simulink model "Simulink_generic_interface_2018b"  (R2018b)
settings: Solver=FixedStepAuto  StartTime=0.0  StopTime=inf  FixedStep=0.0005  RelTol=1e-3
settings Model: Creator=matti  LastModifiedBy=User
settings DataIOCC: ReturnWorkspaceOutputs=on
settings DebuggingCC: UnconnectedInputMsg=none  UnconnectedOutputMsg=none  UnconnectedLineMsg=none
settings ModelReferenceCC: EnableRefExpFcnMdlSchedulingChecks=off
settings RTWCC: Description=Generic Real-Time Target

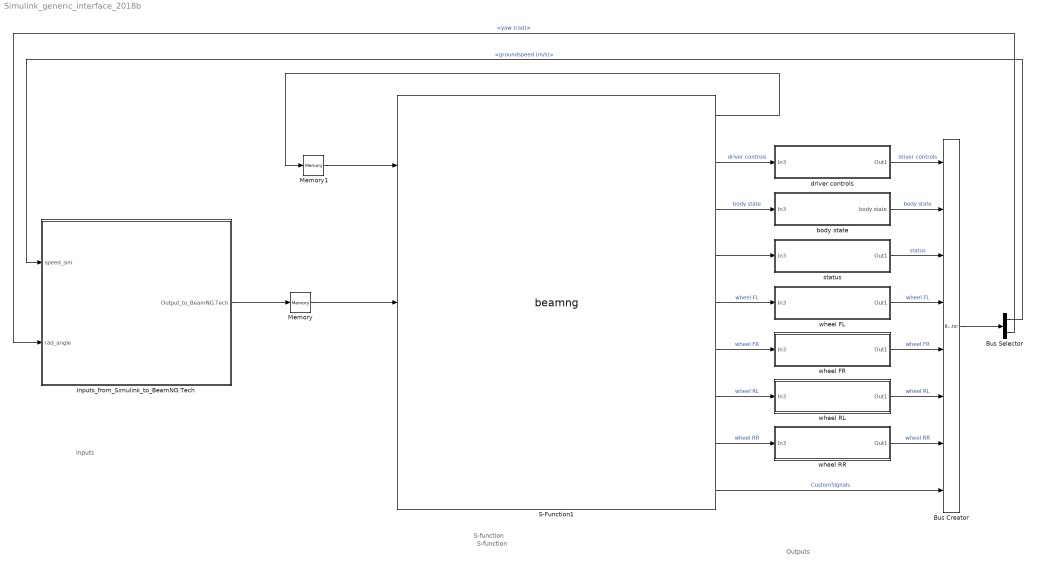
== system Simulink_generic_interface_2018b ==
  note: Inputs
  note: S-function
  note: S-function
  note: Outputs
  Bus Creator : BusCreator  Inputs=8
  Bus Selector : BusSelector  OutputSignals=body state.groundspeed (m/s),body state.yaw (rad)
  Inputs_from_Simulink_to_BeamNG.Tech : Subsystem
  Memory : Memory
  Memory1 : Memory
  S-Function1 : S-Function  FunctionName=beamng  SFunctionDeploymentMode=off  EnableBusSupport=off
      mask Display: image('logo_beamng1.png')
  body state : Subsystem
  driver controls : Subsystem
  status : Subsystem
  wheel FL : Subsystem
  wheel FR : Subsystem
  wheel RL : Subsystem
  wheel RR : Subsystem
  wires:
  S-Function1/3 -> body state/1(In3)  "body state"
  S-Function1/9 -> Bus Creator/8  "CustomSignals"
  S-Function1/5 -> wheel FL/1(In3)  "wheel FL"
  S-Function1/6 -> wheel FR/1(In3)  "wheel FR"
  S-Function1/7 -> wheel RL/1(In3)  "wheel RL"
  S-Function1/8 -> wheel RR/1(In3)  "wheel RR"
  S-Function1/2 -> driver controls/1(In3)  "driver controls"
  Bus Creator/1 -> Bus Selector/1
  Bus Selector/1 -> Inputs_from_Simulink_to_BeamNG.Tech/1(speed_sim)  "<groundspeed (m/s)>"
  Bus Selector/2 -> Inputs_from_Simulink_to_BeamNG.Tech/2(rad_angle)  "<yaw (rad)>"
  driver controls/1(Out1) -> Bus Creator/1  "driver controls"
  body state/1(body state) -> Bus Creator/2  "body state"
  status/1(Out1) -> Bus Creator/3  "status"
  wheel FL/1(Out1) -> Bus Creator/4  "wheel FL"
  wheel FR/1(Out1) -> Bus Creator/5  "wheel FR"
  wheel RL/1(Out1) -> Bus Creator/6  "wheel RL"
  wheel RR/1(Out1) -> Bus Creator/7  "wheel RR"
  Memory/1 -> S-Function1/2
  Inputs_from_Simulink_to_BeamNG.Tech/1(Output_to_BeamNG.Tech) -> Memory/1
  Memory1/1 -> S-Function1/1
  S-Function1/1 -> Memory1/1
  S-Function1/4 -> status/1(In3)

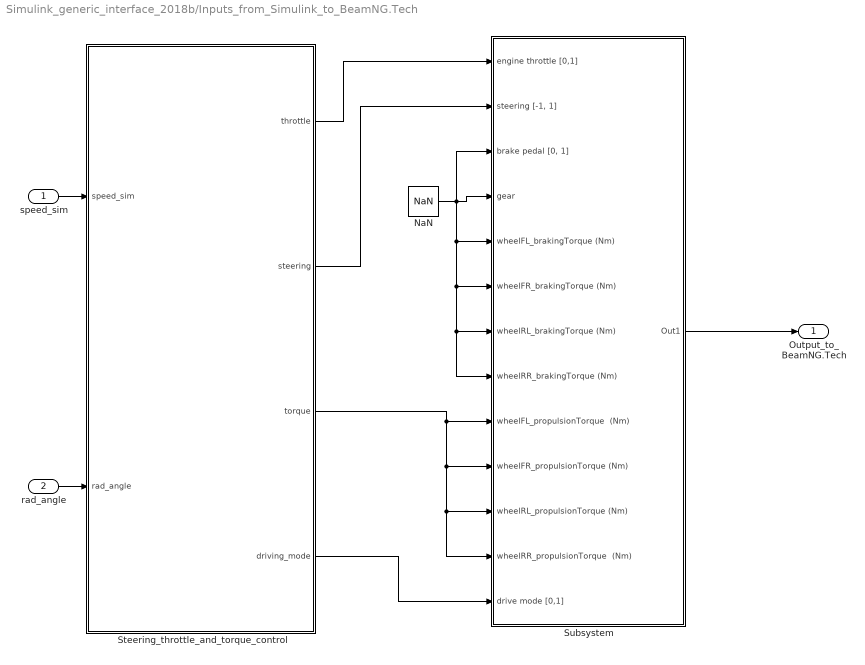
== system Simulink_generic_interface_2018b/Inputs_from_Simulink_to_BeamNG.Tech ==
  speed_sim : Inport
  rad_angle : Inport  Port=2
  NaN : Constant  Value=NaN  OutDataTypeStr=Inherit: Inherit via back propagation
  Steering_throttle_and_torque_control : Subsystem
  Subsystem : Subsystem
  Output_to_BeamNG.Tech : Outport  VectorParamsAs1DForOutWhenUnconnected=on
  wires:
  rad_angle/1 -> Steering_throttle_and_torque_control/2(rad_angle)
  Subsystem/1(Out1) -> Output_to_BeamNG.Tech/1
  speed_sim/1 -> Steering_throttle_and_torque_control/1(speed_sim)
  Steering_throttle_and_torque_control/3(torque) -> Subsystem/10(wheelFR_propulsionTorque (Nm)), Subsystem/11(wheelRL_propulsionTorque (Nm)), Subsystem/12(wheelRR_propulsionTorque	 (Nm)), Subsystem/9(wheelFL_propulsionTorque	 (Nm))
  Steering_throttle_and_torque_control/4(driving_mode) -> Subsystem/13(drive mode [0,1])
  Steering_throttle_and_torque_control/2(steering) -> Subsystem/2("steering\t[-1, 1]")
  Steering_throttle_and_torque_control/1(throttle) -> Subsystem/1("engine throttle [0,1] ")
  NaN/1 -> Subsystem/3("brake pedal [0, 1]"), Subsystem/8("wheelRR_brakingTorque (Nm)\t"), Subsystem/7("wheelRL_brakingTorque (Nm)\t"), Subsystem/6("wheelFR_brakingTorque (Nm)\t"), Subsystem/5("wheelFL_brakingTorque (Nm)\t"), Subsystem/4("gear ")

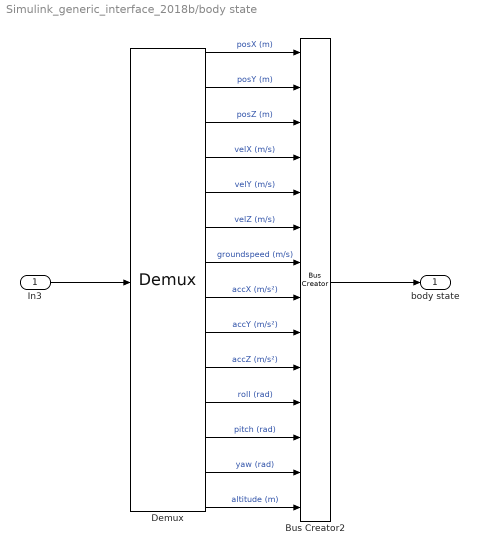
== system Simulink_generic_interface_2018b/body state ==
  In3 : Inport
  Bus Creator2 : BusCreator  Inputs=14
  Demux : Demux  Outputs=14
  body state : Outport  VectorParamsAs1DForOutWhenUnconnected=on
  wires:
  In3/1 -> Demux/1
  Demux/1 -> Bus Creator2/1  "posX (m)"
  Demux/2 -> Bus Creator2/2  "posY (m)"
  Demux/3 -> Bus Creator2/3  "posZ (m)"
  Demux/4 -> Bus Creator2/4  "velX (m/s)"
  Demux/5 -> Bus Creator2/5  "velY (m/s)"
  Demux/6 -> Bus Creator2/6  "velZ (m/s)"
  Demux/7 -> Bus Creator2/7  "groundspeed (m/s)"
  Demux/8 -> Bus Creator2/8  "accX (m/s²)"
  Demux/9 -> Bus Creator2/9  "accY (m/s²)"
  Demux/10 -> Bus Creator2/10  "accZ (m/s²)"
  Demux/11 -> Bus Creator2/11  "roll (rad)"
  Demux/12 -> Bus Creator2/12  "pitch (rad)"
  Demux/13 -> Bus Creator2/13  "yaw (rad)"
  Demux/14 -> Bus Creator2/14  "altitude (m)"
  Bus Creator2/1 -> body state/1

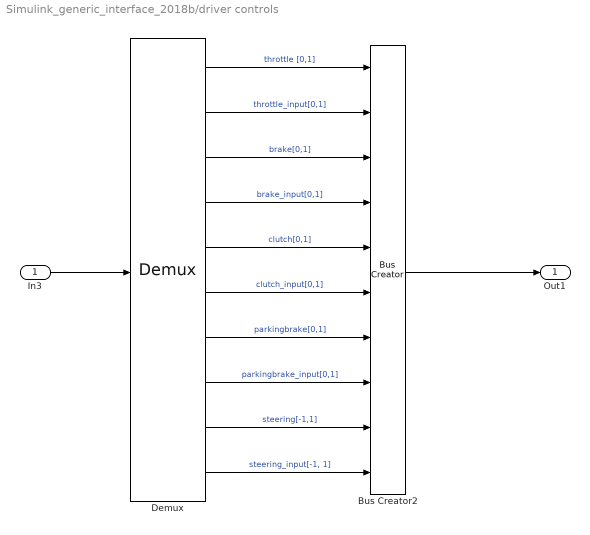
== system Simulink_generic_interface_2018b/driver controls ==
  In3 : Inport
  Bus Creator2 : BusCreator  Inputs=10
  Demux : Demux  Outputs=10
  Out1 : Outport  VectorParamsAs1DForOutWhenUnconnected=on
  wires:
  In3/1 -> Demux/1
  Demux/1 -> Bus Creator2/1  "throttle [0,1]"
  Demux/2 -> Bus Creator2/2  "throttle_input[0,1]"
  Demux/3 -> Bus Creator2/3  "brake[0,1]"
  Demux/4 -> Bus Creator2/4  "brake_input[0,1]"
  Demux/5 -> Bus Creator2/5  "clutch[0,1]"
  Demux/6 -> Bus Creator2/6  "clutch_input[0,1]"
  Demux/7 -> Bus Creator2/7  "parkingbrake[0,1]"
  Demux/8 -> Bus Creator2/8  "parkingbrake_input[0,1]"
  Demux/9 -> Bus Creator2/9  "steering[-1,1]"
  Demux/10 -> Bus Creator2/10  "steering_input[-1, 1]"
  Bus Creator2/1 -> Out1/1

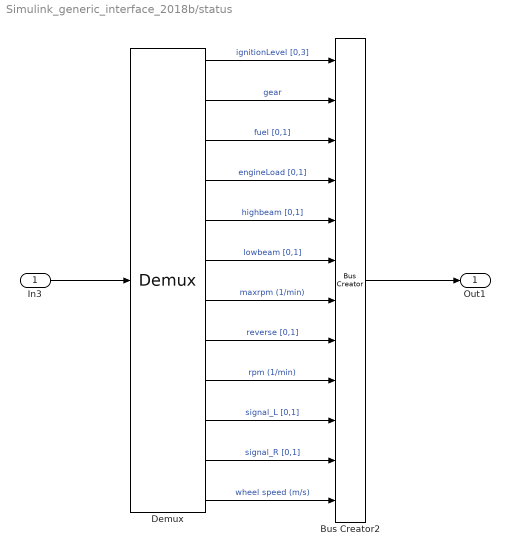
== system Simulink_generic_interface_2018b/status ==
  In3 : Inport
  Bus Creator2 : BusCreator  Inputs=12
  Demux : Demux  Outputs=12
  Out1 : Outport  VectorParamsAs1DForOutWhenUnconnected=on
  wires:
  Demux/12 -> Bus Creator2/12  "wheel speed (m/s)"
  Demux/11 -> Bus Creator2/11  "signal_R [0,1]"
  Demux/10 -> Bus Creator2/10  "signal_L [0,1]"
  Demux/9 -> Bus Creator2/9  "rpm (1/min)"
  Demux/8 -> Bus Creator2/8  "reverse [0,1]"
  Demux/7 -> Bus Creator2/7  "maxrpm (1/min)"
  Demux/6 -> Bus Creator2/6  "lowbeam [0,1]"
  Demux/5 -> Bus Creator2/5  "highbeam [0,1]"
  Demux/4 -> Bus Creator2/4  "engineLoad [0,1]"
  Demux/3 -> Bus Creator2/3  "fuel [0,1]"
  Demux/2 -> Bus Creator2/2  "gear"
  Demux/1 -> Bus Creator2/1  "ignitionLevel [0,3]"
  In3/1 -> Demux/1
  Bus Creator2/1 -> Out1/1

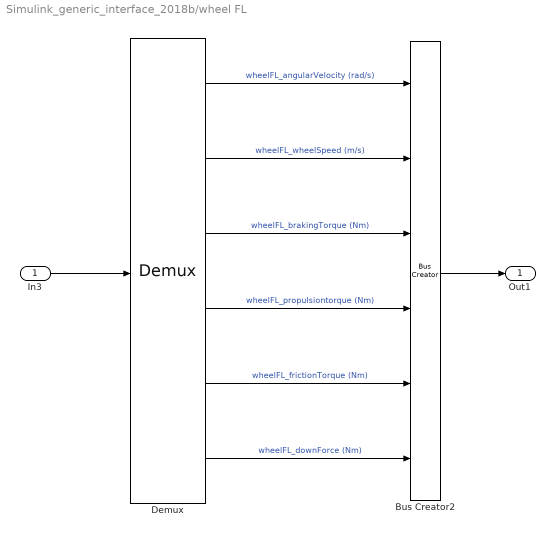
== system Simulink_generic_interface_2018b/wheel FL ==
  In3 : Inport
  Bus Creator2 : BusCreator  Inputs=6
  Demux : Demux  Outputs=6
  Out1 : Outport  VectorParamsAs1DForOutWhenUnconnected=on
  wires:
  In3/1 -> Demux/1
  Demux/1 -> Bus Creator2/1  "wheelFL_angularVelocity (rad/s)"
  Demux/2 -> Bus Creator2/2  "wheelFL_wheelSpeed (m/s)"
  Demux/3 -> Bus Creator2/3  "wheelFL_brakingTorque (Nm)"
  Demux/4 -> Bus Creator2/4  "wheelFL_propulsiontorque (Nm)"
  Demux/5 -> Bus Creator2/5  "wheelFL_frictionTorque (Nm)"
  Demux/6 -> Bus Creator2/6  "wheelFL_downForce (Nm)"
  Bus Creator2/1 -> Out1/1

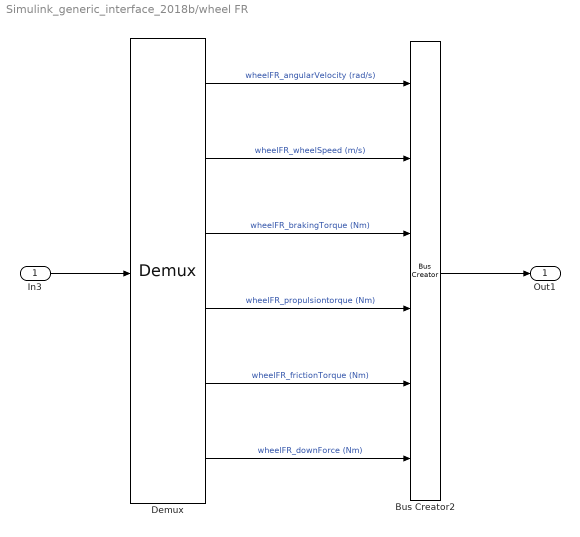
== system Simulink_generic_interface_2018b/wheel FR ==
  In3 : Inport
  Bus Creator2 : BusCreator  Inputs=6
  Demux : Demux  Outputs=6
  Out1 : Outport  VectorParamsAs1DForOutWhenUnconnected=on
  wires:
  Demux/6 -> Bus Creator2/6  "wheelFR_downForce (Nm)"
  Demux/5 -> Bus Creator2/5  "wheelFR_frictionTorque (Nm)"
  Demux/4 -> Bus Creator2/4  "wheelFR_propulsiontorque (Nm)"
  Demux/3 -> Bus Creator2/3  "wheelFR_brakingTorque (Nm)"
  Demux/2 -> Bus Creator2/2  "wheelFR_wheelSpeed (m/s)"
  Demux/1 -> Bus Creator2/1  "wheelFR_angularVelocity (rad/s)"
  In3/1 -> Demux/1
  Bus Creator2/1 -> Out1/1

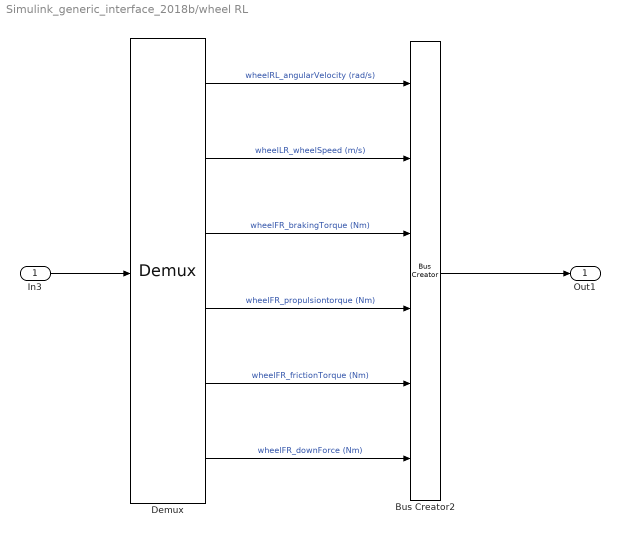
== system Simulink_generic_interface_2018b/wheel RL ==
  In3 : Inport
  Bus Creator2 : BusCreator  Inputs=6
  Demux : Demux  Outputs=6
  Out1 : Outport  VectorParamsAs1DForOutWhenUnconnected=on
  wires:
  In3/1 -> Demux/1
  Demux/1 -> Bus Creator2/1  "wheelRL_angularVelocity (rad/s)"
  Demux/2 -> Bus Creator2/2  "wheelLR_wheelSpeed (m/s)"
  Demux/3 -> Bus Creator2/3  "wheelFR_brakingTorque (Nm)"
  Demux/4 -> Bus Creator2/4  "wheelFR_propulsiontorque (Nm)"
  Demux/5 -> Bus Creator2/5  "wheelFR_frictionTorque (Nm)"
  Demux/6 -> Bus Creator2/6  "wheelFR_downForce (Nm)"
  Bus Creator2/1 -> Out1/1

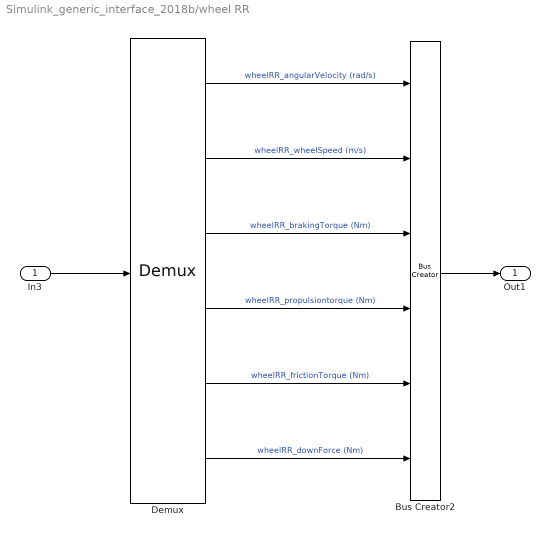
== system Simulink_generic_interface_2018b/wheel RR ==
  In3 : Inport
  Bus Creator2 : BusCreator  Inputs=6
  Demux : Demux  Outputs=6
  Out1 : Outport  VectorParamsAs1DForOutWhenUnconnected=on
  wires:
  Demux/6 -> Bus Creator2/6  "wheelRR_downForce (Nm)"
  Demux/5 -> Bus Creator2/5  "wheelRR_frictionTorque (Nm)"
  Demux/4 -> Bus Creator2/4  "wheelRR_propulsiontorque (Nm)"
  Demux/3 -> Bus Creator2/3  "wheelRR_brakingTorque (Nm)"
  Demux/2 -> Bus Creator2/2  "wheelRR_wheelSpeed (m/s)"
  Demux/1 -> Bus Creator2/1  "wheelRR_angularVelocity (rad/s)"
  In3/1 -> Demux/1
  Bus Creator2/1 -> Out1/1

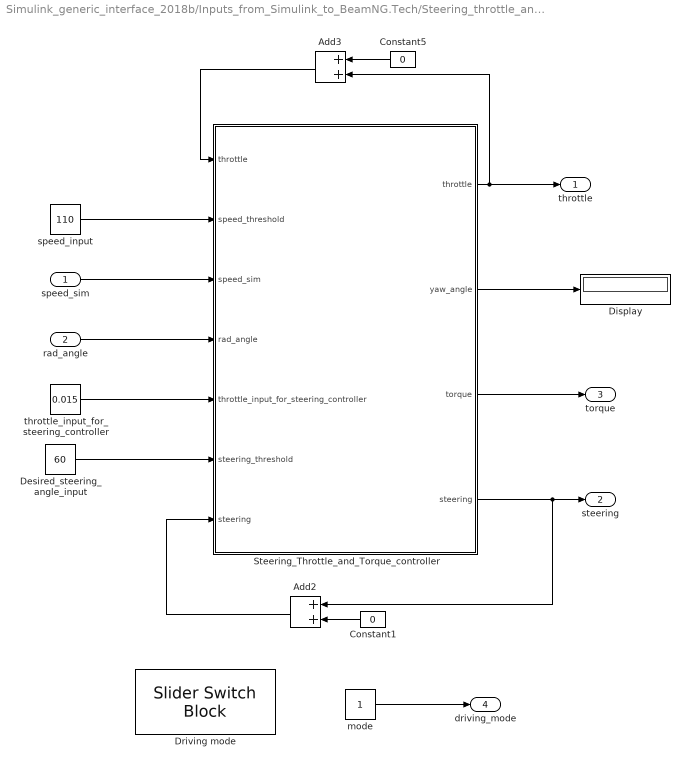
== system Simulink_generic_interface_2018b/Inputs_from_Simulink_to_BeamNG.Tech/Steering_throttle_and_torque_control ==
  speed_sim : Inport
  rad_angle : Inport  Port=2
  Add2 : Sum
  Add3 : Sum
  Constant1 : Constant  Value=0
  Constant5 : Constant  Value=0
  Desired_steering_angle_input : Constant  Value=60
  Display : Display
  Driving mode : SliderSwitchBlock  WebBlockId=467
      settings: Values={{'Torque', 'Pedal'}, [1 0]}
  Steering_Throttle_and_Torque_controller : MATLAB Function  TreatAsAtomicUnit=on
  mode : Constant
  speed_input : Constant  Value=110
  throttle_input_for_steering_controller : Constant  Value=0.015
  throttle : Outport  VectorParamsAs1DForOutWhenUnconnected=on
  steering : Outport  Port=2  VectorParamsAs1DForOutWhenUnconnected=on
  torque : Outport  Port=3  VectorParamsAs1DForOutWhenUnconnected=on
  driving_mode : Outport  Port=4  VectorParamsAs1DForOutWhenUnconnected=on
  wires:
  speed_input/1 -> Steering_Throttle_and_Torque_controller/2(speed_threshold)
  Desired_steering_angle_input/1 -> Steering_Throttle_and_Torque_controller/6(steering_threshold)
  Constant5/1 -> Add3/1
  Steering_Throttle_and_Torque_controller/1(throttle) -> Add3/2, throttle/1
  Add2/1 -> Steering_Throttle_and_Torque_controller/7("steering ")
  Constant1/1 -> Add2/2
  Add3/1 -> Steering_Throttle_and_Torque_controller/1("throttle ")
  mode/1 -> driving_mode/1
  Steering_Throttle_and_Torque_controller/3(torque) -> torque/1
  Steering_Throttle_and_Torque_controller/4(steering) -> Add2/1, steering/1
  rad_angle/1 -> Steering_Throttle_and_Torque_controller/4(rad_angle)
  speed_sim/1 -> Steering_Throttle_and_Torque_controller/3(speed_sim)
  throttle_input_for_steering_controller/1 -> Steering_Throttle_and_Torque_controller/5(throttle_input_for_steering_controller)
  Steering_Throttle_and_Torque_controller/2(yaw_angle) -> Display/1

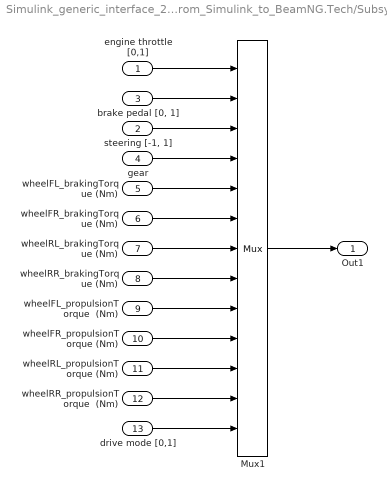
== system Simulink_generic_interface_2018b/Inputs_from_Simulink_to_BeamNG.Tech/Subsystem ==
  "engine throttle [0,1] " : Inport
  "steering\t[-1, 1]" : Inport  Port=2
  "brake pedal [0, 1]" : Inport  Port=3
  "gear " : Inport  Port=4
  "wheelFL_brakingTorque (Nm)\t" : Inport  Port=5
  "wheelFR_brakingTorque (Nm)\t" : Inport  Port=6
  "wheelRL_brakingTorque (Nm)\t" : Inport  Port=7
  "wheelRR_brakingTorque (Nm)\t" : Inport  Port=8
  wheelFL_propulsionTorque	 (Nm) : Inport  Port=9
  wheelFR_propulsionTorque (Nm) : Inport  Port=10
  wheelRL_propulsionTorque (Nm) : Inport  Port=11
  wheelRR_propulsionTorque	 (Nm) : Inport  Port=12
  drive mode [0,1] : Inport  Port=13
  Mux1 : Mux  Inputs=13
  Out1 : Outport  VectorParamsAs1DForOutWhenUnconnected=on
  wires:
  "wheelFR_brakingTorque (Nm)\t"/1 -> Mux1/6
  "wheelRL_brakingTorque (Nm)\t"/1 -> Mux1/7
  "wheelRR_brakingTorque (Nm)\t"/1 -> Mux1/8
  "brake pedal [0, 1]"/1 -> Mux1/2
  drive mode [0,1]/1 -> Mux1/13
  wheelRR_propulsionTorque	 (Nm)/1 -> Mux1/12
  wheelFR_propulsionTorque (Nm)/1 -> Mux1/10
  wheelRL_propulsionTorque (Nm)/1 -> Mux1/11
  "wheelFL_brakingTorque (Nm)\t"/1 -> Mux1/5
  "engine throttle [0,1] "/1 -> Mux1/1
  "gear "/1 -> Mux1/4
  "steering\t[-1, 1]"/1 -> Mux1/3
  wheelFL_propulsionTorque	 (Nm)/1 -> Mux1/9
  Mux1/1 -> Out1/1

== matlab function Simulink_generic_interface_2018b/Inputs_from_Simulink_to_BeamNG.Tech/Steering_throttle_and_torque_control/Steering_Throttle_and_Torque_controller ==
  data: throttle input; throttle output; yaw_angle output; torque output; steering output; speed_threshold input; speed_sim input; rad_angle input; throttle_input_for_steering_controller input; steering_threshold input; steering input
function [throttle,yaw_angle,torque,steering]= Controller(throttle,speed_threshold,speed_sim,rad_angle,throttle_input_for_steering_controller,steering_threshold,steering)
    % Steering 
    steering_clearance=1; % in degrees
    % here's converting the angle from radiant to degree      
    yaw_angle=rad_angle*(180/pi);
    if yaw_angle <= (steering_threshold-steering_clearance)
    steering=-throttle_input_for_steering_controller;
    end   

    if  yaw_angle > (steering_threshold)
    steering=throttle_input_for_steering_controller;
    end   


    % Throttle and Torque 
    speed_clearance=10;
    actual_speed=speed_sim*3.6;
    if actual_speed <= 5
    torque = 270 ; 
    throttle=0.5;
    elseif actual_speed <= (speed_threshold-speed_clearance)
    throttle=0.5;
    torque = 200 ; 
    elseif  actual_speed > (speed_threshold)
    throttle=-0.05;
    torque = 65; 
    else
    torque = 170; 
    end
    end
